simulink model "Task5"  (R2022a)
settings: Solver=FixedStepAuto  StartTime=0.0  StopTime=10  FixedStep=0.0001  RelTol=1e-3
undefined symbols (not defined in the file): A, a_0, a_1, a_2, a_3, s1, s2, s3, s4
settings Model: Creator=Family  LastModifiedBy=Family

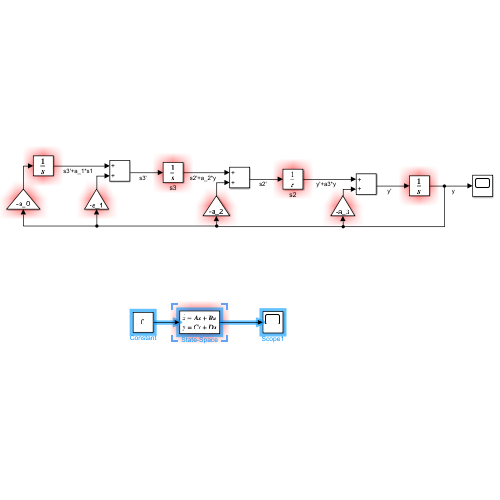
[thumbnail: Simulink's stored preview of the top-level diagram]
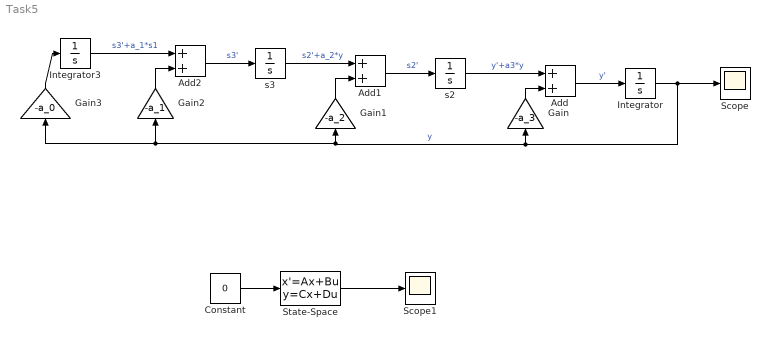
== system Task5 ==
  Add : Sum
  Add1 : Sum
  Add2 : Sum
  Constant : Constant  Value=0
  Gain : Gain  Gain=-a_3
  Gain1 : Gain  Gain=-a_2
  Gain2 : Gain  Gain=-a_1
  Gain3 : Gain  Gain=-a_0
  Integrator : Integrator  InitialCondition=s1
  Integrator3 : Integrator  InitialCondition=s4
  Scope : Scope
  Scope1 : Scope
  State-Space : StateSpace  A=A  B=[0;0;0;0]  C=[1 0 1 0]  D=0  InitialCondition=[1;0;1;0]
  s2 : Integrator  InitialCondition=s2
  s3 : Integrator  InitialCondition=s3
  wires:
  Integrator/1 -> Gain3/1, Gain2/1, Gain1/1, Gain/1, Scope/1  "y"
  Add/1 -> Integrator/1  "y'"
  Gain/1 -> Add/2
  s2/1 -> Add/1  "y'+a3*y"
  Add1/1 -> s2/1  "s2'"
  Gain1/1 -> Add1/2
  s3/1 -> Add1/1  "s2'+a_2*y"
  Add2/1 -> s3/1  "s3'"
  Gain2/1 -> Add2/2
  Integrator3/1 -> Add2/1  "s3'+a_1*s1"
  Gain3/1 -> Integrator3/1
  Constant/1 -> State-Space/1
  State-Space/1 -> Scope1/1
